simulink model "pid"  (R2020b)
settings: Solver=VariableStepAuto  StartTime=0.0  StopTime=10.0  RelTol=1e-3
undefined symbols (not defined in the file): Kd, Ki, Kp, N
settings Model: Creator=stkaravind  LastModifiedBy=stkaravind

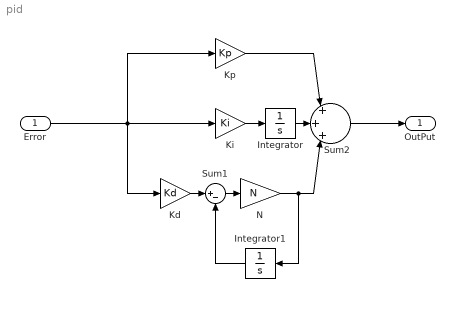
== system pid ==
  Error : Inport  OutDataTypeStr=double  PortDimensions=1  SampleTime=0
  Integrator : Integrator
  Integrator1 : Integrator
  Kd : Gain  Gain=Kd
  Ki : Gain  Gain=Ki
  Kp : Gain  Gain=Kp
  N : Gain  Gain=N
  Sum1 : Sum  Inputs=|+-
  Sum2 : Sum  Inputs=|+|+|+|
  OutPut : Outport  OutDataTypeStr=double  PortDimensions=1  SampleTime=0
  wires:
  Kd/1 -> Sum1/1
  Kp/1 -> Sum2/1
  Ki/1 -> Integrator/1
  Integrator/1 -> Sum2/2
  Integrator1/1 -> Sum1/2
  N/1 -> Sum2/3, Integrator1/1
  Error/1 -> Kd/1, Kp/1, Ki/1
  Sum1/1 -> N/1
  Sum2/1 -> OutPut/1
